simulink library "AnnVncBtc"  (R2022b)
settings: Solver=VariableStepAuto  StartTime=0.0  StopTime=10.0  RelTol=1e-3
libraries: FeaturePath x1, HandyTextFile x1
settings Model: Creator=kl13806  LastModifiedBy=kl13806
settings SolverCC: AlgebraicLoopSolver=TrustRegion
settings DebuggingCC: UnconnectedInputMsg=warning  UnconnectedOutputMsg=warning  UnconnectedLineMsg=warning  SFMachineParentedDataDiag=warning
settings ModelReferenceCC: EnableRefExpFcnMdlSchedulingChecks=on
settings RTWCC: DLArmComputeVersion=19.05

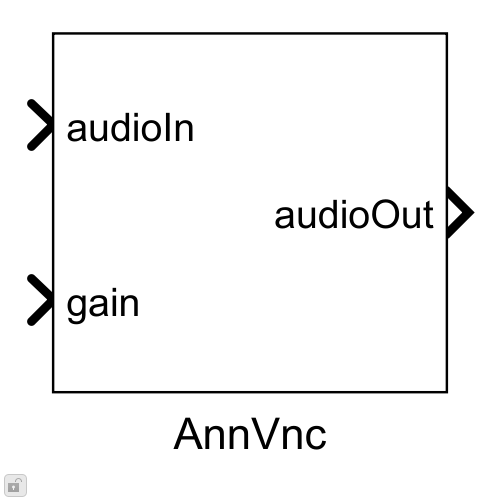
[thumbnail: Simulink's stored preview of the top-level diagram]
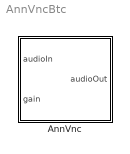
== system AnnVncBtc ==
  AnnVnc : Subsystem  mask(Blocklib AnnVnc){Config=[], FeatureName=VNC}
      mask prompts: Config "AnnVncConfig"; FeatureName "Feature path name:"
      mask init:
      | blkh=gcbh;
      | Config=BTConfig.Assert(blkh,Config);
      | Config.Validate();
      | 
      | BTConfig.InitSetFeatureIfPresent(blkh,'FeatureName');
      mask Callback Config: BTConfig.CallbackHideIfPresent(gcbh,{'FeatureName'});
      mask TypeOptions FeatureName: FeaturePath/FeatureName

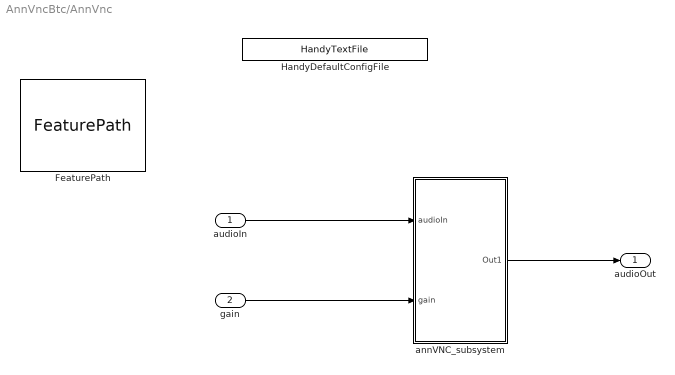
== system AnnVncBtc/AnnVnc ==
  audioIn : Inport
  gain : Inport  Port=2
  FeaturePath : FeaturePath/FeaturePath  FeatureName=VNC  IsGroup=off  GroupNumber=-1  IsModule=off  TriggerInit=[210 89 335 181]
  HandyDefaultConfigFile : HandyTextFile/HandyTextFile  TemplateSource=Config  FileSuffix=Init  OpenDialogOnLoad=off  UseThisBlockName=off  TheDefaultText=|  ShowInLibBrowser=on
      | % $(FILENAME) Setup model parameters for each "Init" callback (e.g. update diagram)
      | sample_rate_in_hertz = 44100;
      | frame_size = 32;
      | sysin_channel_count = 2;
  annVNC_subsystem : Subsystem
  audioOut : Outport  VectorParamsAs1DForOutWhenUnconnected=off
  wires:
  annVNC_subsystem/1(Out1) -> audioOut/1
  gain/1 -> annVNC_subsystem/2(gain)
  audioIn/1 -> annVNC_subsystem/1(audioIn)

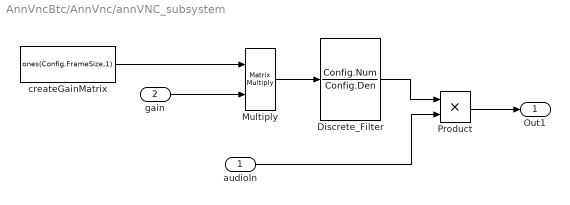
== system AnnVncBtc/AnnVnc/annVNC_subsystem ==
  audioIn : Inport
  gain : Inport  Port=2
  Discrete_Filter : DiscreteFilter  Numerator=Config.Num  Denominator=Config.Den  InitialStates=Config.ZInit  InputProcessing=Columns as channels (frame based)  FilterStructure=Direct form II transposed  a0EqualsOne=on
  Multiply : Product  Multiplication=Matrix(*)
  Product : Product
  createGainMatrix : Constant  Value=ones(Config.FrameSize,1)  VectorParams1D=off  OutDataTypeStr=single
  Out1 : Outport  VectorParamsAs1DForOutWhenUnconnected=off
  wires:
  gain/1 -> Multiply/2
  Product/1 -> Out1/1
  audioIn/1 -> Product/2
  Discrete_Filter/1 -> Product/1
  createGainMatrix/1 -> Multiply/1
  Multiply/1 -> Discrete_Filter/1
